simulink model "Controle_principal"  (R2015a)
settings: Solver=ode3  StartTime=0.0  StopTime=inf  RelTol=1e-3
libraries: arduinolib x4
settings Model: SimulationMode=external  ExtModeTrigDuration=2  Creator=kelvin  LastModifiedBy=kelvin
settings OptimizationCC: OptimizeModelRefInitCode=on  LifeSpan=1
settings DebuggingCC: UnderspecifiedInitializationDetection=Classic  MergeDetectMultiDrivingBlocksExec=none
settings HardwareCC: ProdBitPerInt=16  ProdBitPerPointer=8  ProdIntDivRoundTo=Zero  ProdEndianess=LittleEndian  ProdWordSize=8  ProdHWDeviceType=Atmel->AVR
settings RTWCC: SystemTargetFile=realtime.tlc  GenerateMakefile=off  TemplateMakefile=realtime.tmf  Description=Run on Target Hardware  RTWVerbose=off
settings ERTTargetCC: CombineOutputUpdateFcns=off  ExtMode=on  ExtModeTransport=3  ExtModeMexFile=ext_serial_win32_comm_rtt  ExtModeMexArgs=0 7 115200 30  ERTSrcFileBannerTemplate=realtime_code_template.cgt  ERTHdrFileBannerTemplate=realtime_code_template.cgt  ERTDataSrcFileTemplate=realtime_code_template.cgt  ERTDataHdrFileTemplate=realtime_code_template.cgt  ERTCustomFileTemplate=realtime_file_process.tlc

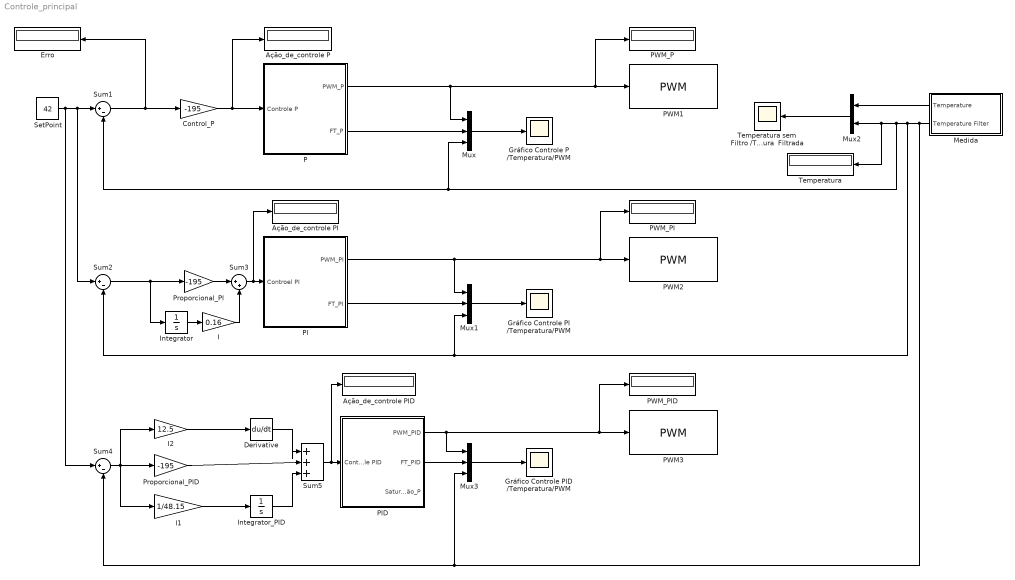
== system Controle_principal ==
  Ação_de_controle P : Display
  Ação_de_controle PI : Display
  Ação_de_controle PID : Display
  Control_P : Gain  Gain=-195
  Derivative : Derivative
  "Erro " : Display
  Gráfico Controle P /Temperatura/PWM : Scope
      settings: TimeRange=600  YMin=-200  YMax=275  MaxDataPoints=1000
  Gráfico Controle PI /Temperatura/PWM : Scope
      settings: TimeRange=850  YMin=-50  YMax=275
  Gráfico Controle PID /Temperatura/PWM : Scope
      settings: TimeRange=6000  YMin=-20  YMax=32.5  SaveName=ScopeData3
  I : Gain  Gain=0.16
  I1 : Gain  Gain=1/48.15
  I2 : Gain  Gain=12.5
  Integrator : Integrator
  Integrator_PID : Integrator
  Medida : Subsystem
  Mux : Mux  Inputs=3
  Mux1 : Mux  Inputs=3
  Mux2 : Mux  Inputs=2
  Mux3 : Mux  Inputs=3
  "P " : Subsystem
  "PI " : Subsystem
  PID : Subsystem
  PWM1 : arduinolib/PWM  pinNumber=9  blockPlatform=arduino
  PWM2 : arduinolib/PWM  pinNumber=10  blockPlatform=arduino
  PWM3 : arduinolib/PWM  pinNumber=8  blockPlatform=arduino
  PWM_P : Display
  PWM_PI : Display
  PWM_PID : Display
  Proporcional_PI : Gain  Gain=-195
  Proporcional_PID : Gain  Gain=-195
  SetPoint : Constant  Value=42
  Sum1 : Sum  Inputs=|+-
  Sum2 : Sum  Inputs=|+-
  Sum3 : Sum  Inputs=|++
  Sum4 : Sum  Inputs=|+-  AccumDataTypeStr=double  OutDataTypeStr=double
  Sum5 : Sum  Inputs=|+++
  "Temperatura " : Display
  Temperatura sem Filtro /Temperatura  Filtrada : Scope
      settings: ShowLegends=on  TimeRange=5000  YMin=28  YMax=42  SaveName=ScopeData2
  wires:
  Mux/1 -> Gráfico Controle P /Temperatura/PWM/1
  Medida/2(Temperature Filter) -> Mux3/3, Sum4/2, Mux1/3, Sum2/2, Sum1/2, Mux/3, "Temperatura "/1, Mux2/2
  "P "/1(PWM_P) -> PWM_P/1, PWM1/1, Mux/1
  "P "/2(FT_P) -> Mux/2
  Control_P/1 -> Ação_de_controle P/1, "P "/1(Controle P)
  Sum1/1 -> "Erro "/1, Control_P/1
  Mux1/1 -> Gráfico Controle PI /Temperatura/PWM/1
  "PI "/2(FT_PI) -> Mux1/2
  "PI "/1(PWM_PI) -> PWM_PI/1, PWM2/1, Mux1/1
  Integrator/1 -> I/1
  Sum3/1 -> Ação_de_controle PI/1, "PI "/1(Controel PI)
  I/1 -> Sum3/2
  Mux2/1 -> Temperatura sem Filtro /Temperatura  Filtrada/1
  Medida/1(Temperature) -> Mux2/1
  Mux3/1 -> Gráfico Controle PID /Temperatura/PWM/1
  PID/2(FT_PID) -> Mux3/2
  SetPoint/1 -> Sum4/1, Sum2/1, Sum1/1
  PID/1(PWM_PID) -> PWM_PID/1, PWM3/1, Mux3/1
  Sum2/1 -> Integrator/1, Proporcional_PI/1
  Proporcional_PI/1 -> Sum3/1
  Sum4/1 -> I1/1, I2/1, Proporcional_PID/1
  Sum5/1 -> Ação_de_controle PID/1, PID/1(Controle PID)
  I2/1 -> Derivative/1
  Derivative/1 -> Sum5/1
  Proporcional_PID/1 -> Sum5/2
  I1/1 -> Integrator_PID/1
  Integrator_PID/1 -> Sum5/3

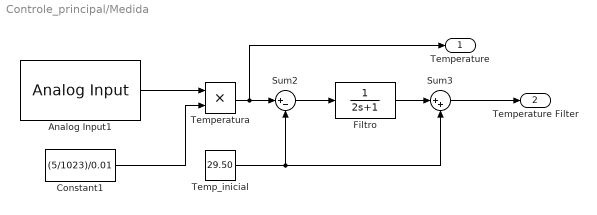
== system Controle_principal/Medida ==
  Analog Input1 : arduinolib/Analog Input  pinNumber=0  sampleTime=0.1  blockPlatform=arduino
  Constant1 : Constant  Value=(5/1023)/0.01  OutDataTypeStr=double
  Filtro : TransferFcn  Denominator=[2 1]
  Sum2 : Sum  Inputs=|+-
  Sum3 : Sum  Inputs=|++
  Temp_inicial : Constant  Value=29.50  VectorParams1D=off  OutDataTypeStr=double
  Temperatura : Product  OutDataTypeStr=double
  Temperature : Outport
  Temperature Filter : Outport  Port=2
  wires:
  Sum3/1 -> Temperature Filter/1
  Analog Input1/1 -> Temperatura/1
  Filtro/1 -> Sum3/1
  Sum2/1 -> Filtro/1
  Temp_inicial/1 -> Sum3/2, Sum2/2
  Constant1/1 -> Temperatura/2
  Temperatura/1 -> Temperature/1, Sum2/1

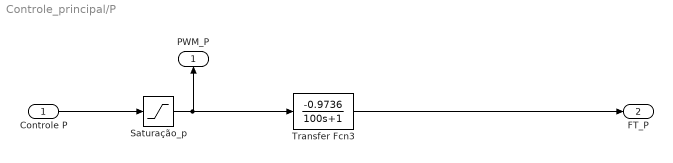
== system Controle_principal/P  ==
  Controle P : Inport
  Saturação_p : Saturate  UpperLimit=255  LowerLimit=20
  Transfer Fcn3 : TransferFcn  Numerator=[-0.9736]  Denominator=[100 1]
  PWM_P : Outport
  FT_P : Outport  Port=2
  wires:
  Saturação_p/1 -> PWM_P/1, Transfer Fcn3/1
  Transfer Fcn3/1 -> FT_P/1
  Controle P/1 -> Saturação_p/1

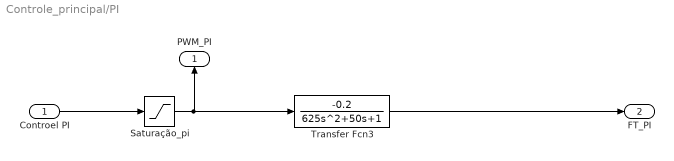
== system Controle_principal/PI  ==
  Controel PI : Inport
  Saturação_pi : Saturate  UpperLimit=255  LowerLimit=20
  Transfer Fcn3 : TransferFcn  Numerator=[-0.2]  Denominator=[625 50 1]
  PWM_PI : Outport
  FT_PI : Outport  Port=2
  wires:
  Controel PI/1 -> Saturação_pi/1
  Transfer Fcn3/1 -> FT_PI/1
  Saturação_pi/1 -> Transfer Fcn3/1, PWM_PI/1

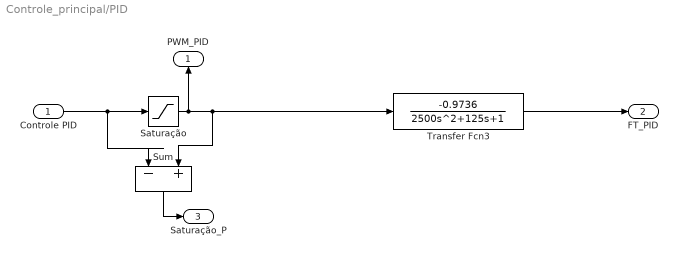
== system Controle_principal/PID ==
  Controle PID : Inport
  Saturação : Saturate  UpperLimit=255  LowerLimit=20
  Sum : Sum  Inputs=|-+
  Transfer Fcn3 : TransferFcn  Numerator=[-0.9736]  Denominator=[2500 125 1]
  PWM_PID : Outport
  FT_PID : Outport  Port=2
  Saturação_P : Outport  Port=3
  wires:
  Saturação/1 -> Sum/2, Transfer Fcn3/1, PWM_PID/1
  Transfer Fcn3/1 -> FT_PID/1
  Controle PID/1 -> Sum/1, Saturação/1
  Sum/1 -> Saturação_P/1
